simulink model "L3_1"  (Simulink 6.0)
settings: Solver=ode45  StartTime=0.0  StopTime=100  RelTol=1e-3
undefined symbols (not defined in the file): kp, Tsum
settings Model: LastModifiedBy=student

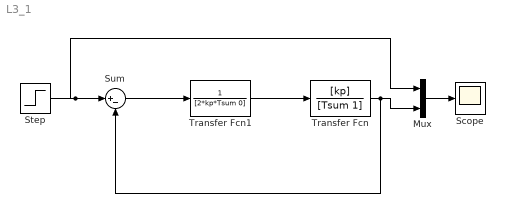
== system L3_1 ==
  Mux : Mux  Inputs=2
  Scope : Scope
  Step : Step  SampleTime=0
  Sum : Sum  Inputs=|+-
  Transfer Fcn : TransferFcn  Numerator=[kp]  Denominator=[Tsum 1]
  Transfer Fcn1 : TransferFcn  Denominator=[2*kp*Tsum 0]
  wires:
  Transfer Fcn1/1 -> Transfer Fcn/1
  Sum/1 -> Transfer Fcn1/1
  Step/1 -> Sum/1, Mux/1
  Mux/1 -> Scope/1
  Transfer Fcn/1 -> Mux/2, Sum/2
